simulink model "AccPed_DrvDemDes"  (R2018a)
settings: configuration reference "cs_ert" (kept outside this file)
values from neighbouring files (symbols this model uses):
  MoFDrDem_trqEng_MAP = 0.0 17.5 36.5 58.9 85.6 117.4 147.9 187.0 215.3 226.2 237.0 244.0 255.8 267.6 279.3 291.1 0.0 7.4 19.8 37.8 62.5 94.5 125.0 165.6 201.1 222.2 236.1 244.0 255.8 267.6 279.3 291.1 0.0 0.8 9.3 23.5 45.9 77.6 108.2 148.1 188.9 216.3 236.1 244.9 256.4 268.0 279.5 291.1 0.0 0.8 1.6 14.7 30.5 60.4 91.6 129.8 173.5 207.4 236.1 244.0 255.8 267.6 279.3 291.1 0.0 0.0 0.0 4.5 17.9 44.2 73.8 111.0 160.3 196.0    [AccPed_DrvDemDes.sldd]
  MoFDrDem_trqEng_MAPX : value not decoded    [AccPed_DrvDemDes.sldd]
  MoFDrDem_trqEng_MAPY : value not decoded    [AccPed_DrvDemDes.sldd]
  SigTst_swtAccPed_C = 0    [AccPed_DrvDemDes.sldd]
  SigTst_trqAccPed_C = 0.0    [AccPed_DrvDemDes.sldd]
undefined symbols (not defined in the file or in its folder): Switch
settings Model: DataDictionary=AccPed_DrvDemDes.sldd  Creator=zhoutinglin  LastModifiedBy=zhoutinglin

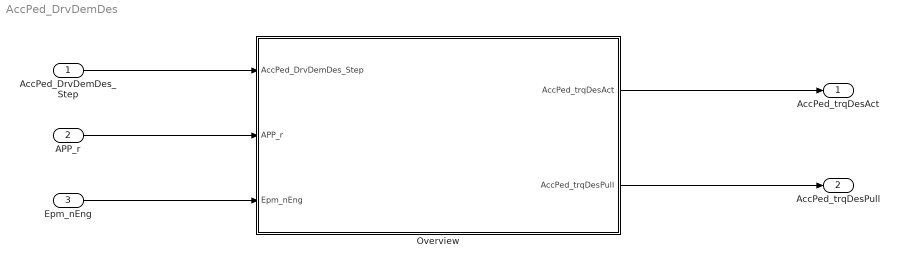
== system AccPed_DrvDemDes ==
  AccPed_DrvDemDes_Step : Inport  OutputFunctionCall=on
  APP_r : Inport  Description=Acceleration pedal sensor 1 value after fault handling  Port=2  OutMin=0  OutMax=100  OutDataTypeStr=Percent  Unit=%  PortDimensions=[1 1]
  Epm_nEng : Inport  Description=Engine speed  Port=3  OutMin=0  OutMax=6000  OutDataTypeStr=ERPM  Unit=rpm  PortDimensions=[1 1]
  Overview : Subsystem
  AccPed_trqDesAct : Outport  Description=driver torque raw of propulsion  OutMin=-3000  OutMax=3000  OutDataTypeStr=Torq  Unit=Nm  PortDimensions=[1 1]
  AccPed_trqDesPull : Outport  Description=Application parameter for driver demand in pull mode for desired value  Port=2  OutMin=-3000  OutMax=3000  OutDataTypeStr=Torq  Unit=Nm  PortDimensions=[1 1]
  wires:
  AccPed_DrvDemDes_Step/1 -> Overview/1(AccPed_DrvDemDes_Step)
  APP_r/1 -> Overview/2(APP_r)
  Epm_nEng/1 -> Overview/3(Epm_nEng)
  Overview/1(AccPed_trqDesAct) -> AccPed_trqDesAct/1
  Overview/2(AccPed_trqDesPull) -> AccPed_trqDesPull/1

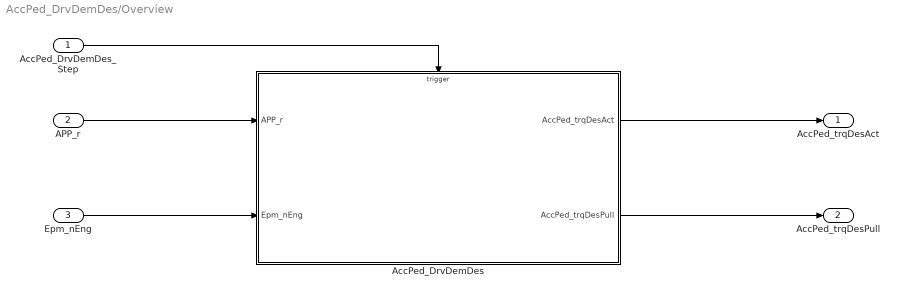
== system AccPed_DrvDemDes/Overview ==
  AccPed_DrvDemDes_Step : Inport
  APP_r : Inport  Port=2
  Epm_nEng : Inport  Port=3
  AccPed_DrvDemDes : Subsystem
  AccPed_trqDesAct : Outport
  AccPed_trqDesPull : Outport  Port=2
  wires:
  APP_r/1 -> AccPed_DrvDemDes/1(APP_r)
  Epm_nEng/1 -> AccPed_DrvDemDes/2(Epm_nEng)
  AccPed_DrvDemDes/1(AccPed_trqDesAct) -> AccPed_trqDesAct/1
  AccPed_DrvDemDes/2(AccPed_trqDesPull) -> AccPed_trqDesPull/1
  AccPed_DrvDemDes_Step/1 -> AccPed_DrvDemDes/Trigger

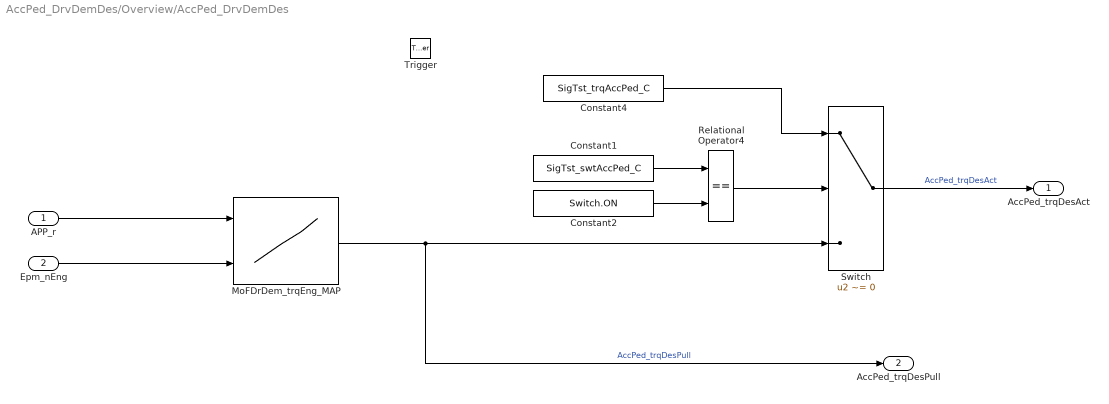
== system AccPed_DrvDemDes/Overview/AccPed_DrvDemDes ==
  APP_r : Inport  Tag=%
  Epm_nEng : Inport  Tag=rpm  Port=2
  Trigger : TriggerPort  TriggerType=function-call  VariantControl=Variant  PortDimensions=1
  Constant1 : Constant  Value=SigTst_swtAccPed_C
  Constant2 : Constant  Value=Switch.ON  OutDataTypeStr=Inherit: Inherit via back propagation
  Constant4 : Constant  Value=SigTst_trqAccPed_C
  MoFDrDem_trqEng_MAP : Lookup_n-D  BreakpointsForDimension1=MoFDrDem_trqEng_MAPY  BreakpointsForDimension2=MoFDrDem_trqEng_MAPX  IndexSearchMethod=Linear search  BeginIndexSearchUsingPreviousIndexResult=on  Table=MoFDrDem_trqEng_MAP  ExtrapMethod=Clip  UseLastTableValue=on  InternalRulePriority=Speed  OutDataTypeStr=Inherit: Inherit via back propagation  SaturateOnIntegerOverflow=on
  Relational Operator4 : RelationalOperator  Operator===  OutDataTypeStr=boolean  RndMeth=Simplest  InputSameDT=on
  Switch : Switch  Criteria=u2 ~= 0  InputSameDT=on
  AccPed_trqDesAct : Outport  Tag=Nm
  AccPed_trqDesPull : Outport  Tag=Nm  Port=2
  wires:
  MoFDrDem_trqEng_MAP/1 -> AccPed_trqDesPull/1, Switch/3  "AccPed_trqDesPull"
  Switch/1 -> AccPed_trqDesAct/1  "AccPed_trqDesAct"
  Relational Operator4/1 -> Switch/2
  Constant2/1 -> Relational Operator4/2
  Constant1/1 -> Relational Operator4/1
  Constant4/1 -> Switch/1
  APP_r/1 -> MoFDrDem_trqEng_MAP/1
  Epm_nEng/1 -> MoFDrDem_trqEng_MAP/2
